simulink model "supercaps_dcbus_control"  (Simulink 7.2)
settings: Solver=ode45  StartTime=0.0  StopTime=5  RelTol=1e-5
undefined symbols (not defined in the file): C_dc, C_sto, K_i, K_v, L, T_i, T_v, V_dc0, V_dc_set, V_sto0
libraries: simulink x3
settings Model: Creator=Pierre  LastModifiedBy=Pierre

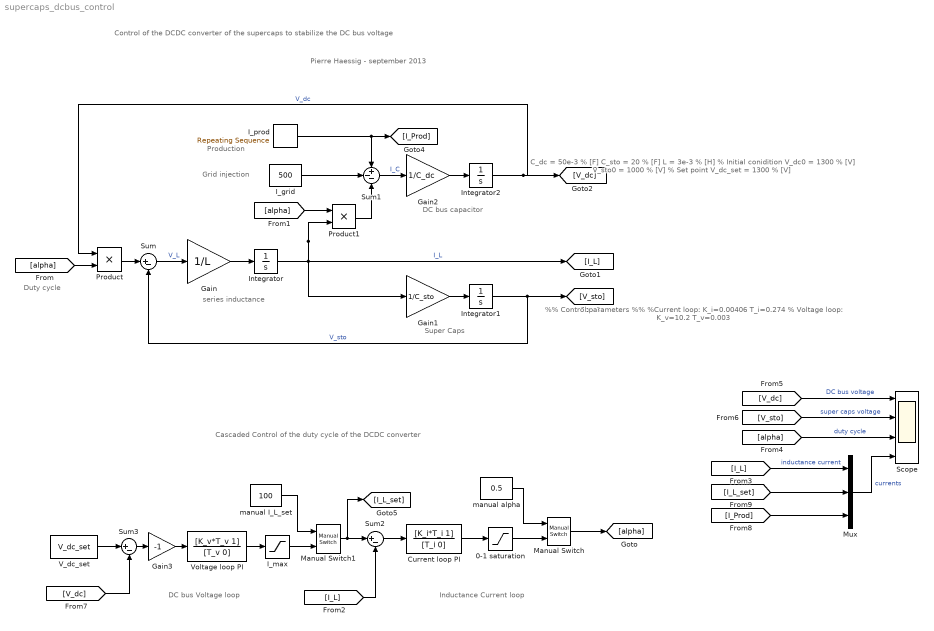
== system supercaps_dcbus_control ==
  note: Control of the DCDC converter of the supercaps
      | to stabilize the DC bus voltage
  note: Production
  note: C_dc = 50e-3 % [F]
      | C_sto = 20 % [F]
      | L = 3e-3 % [H]
      |
      | % Initial conidition
      | V_dc0 = 1300 % [V]
      | V_sto0 = 1000 % [V]
      |
      | % Set point
      | V_dc_set = 1300 % [V]
  note: Grid injection
  note: Cascaded Control
      | of the duty cycle of the DCDC converter
  note: DC bus capacitor
  note: Super Caps
  note: series inductance
  note: Pierre Haessig - september 2013
  note: %% Control parameters %%
      | %Current loop:
      | K_i=0.00406
      | T_i=0.274
      | % Voltage loop:
      | K_v=10.2
      | T_v=0.003
  note: Duty cycle
  note: DC bus Voltage loop
  note: Inductance Current loop
  0-1 saturation : Saturate  UpperLimit=1  LowerLimit=0  OutDataType=sfix(16)  OutScaling=2^0
  Current loop PI : TransferFcn  Numerator=[K_i*T_i 1]  Denominator=[T_i 0]
  Gain : Gain  Gain=1/L  ParameterDataType=sfix(16)  ParameterScaling=2^0  OutDataType=sfix(16)  OutScaling=2^0
  Gain1 : Gain  Gain=1/C_sto  ParameterDataType=sfix(16)  ParameterScaling=2^0  OutDataType=sfix(16)  OutScaling=2^0
  Gain2 : Gain  Gain=1/C_dc  ParameterDataType=sfix(16)  ParameterScaling=2^0  OutDataType=sfix(16)  OutScaling=2^0
  Gain3 : Gain  Gain=-1  ParameterDataType=sfix(16)  ParameterScaling=2^0  OutDataType=sfix(16)  OutScaling=2^0
  I_grid : Constant  Value=500  OutDataType=sfix(16)  OutScaling=2^0
  I_max : Saturate  UpperLimit=1000  LowerLimit=-1000  OutDataType=sfix(16)  OutScaling=2^0
  I_prod : simulink/Sources/Repeating Sequence  SystemSampleTime=-1  rep_seq_t=[0 2 4]  rep_seq_y=[0 1000 0]
  Integrator : Integrator
  Integrator1 : Integrator  InitialCondition=V_sto0
  Integrator2 : Integrator  InitialCondition=V_dc0
  Manual Switch : simulink/Signal Routing/Manual Switch  SystemSampleTime=-1  sw=0  action=0  varsize=off
  Manual Switch1 : simulink/Signal Routing/Manual Switch  SystemSampleTime=-1  sw=0  action=0  varsize=off
  Mux : Mux  Inputs=3
  Product : Product  OutDataType=sfix(16)  OutScaling=2^0  RndMeth=Zero
  Product1 : Product  OutDataType=sfix(16)  OutScaling=2^0  RndMeth=Zero
  Scope : Scope  NumInputPorts=4
      settings: TimeRange=10  YMin=1000~960~-0.5~-4000  YMax=3000~1040~1.5~4000
  Sum : Sum  Inputs=|+-  OutDataType=sfix(16)  OutScaling=2^0
  Sum1 : Sum  Inputs=+--  OutDataType=sfix(16)  OutScaling=2^0
  Sum2 : Sum  Inputs=|+-  OutDataType=sfix(16)  OutScaling=2^0
  Sum3 : Sum  Inputs=|+-  OutDataType=sfix(16)  OutScaling=2^0
  V_dc_set : Constant  Value=V_dc_set  OutDataType=sfix(16)  OutScaling=2^0
  Voltage loop PI : TransferFcn  Numerator=[K_v*T_v 1]  Denominator=[T_v 0]
  manual I_L_set : Constant  Value=100  OutDataType=sfix(16)  OutScaling=2^0
  manual alpha : Constant  Value=0.5  OutDataType=sfix(16)  OutScaling=2^0
  wires:
  Gain/1 -> Integrator/1
  Gain1/1 -> Integrator1/1
  Gain2/1 -> Integrator2/1
  Integrator1/1 -> Sum/2, [V_sto]  "V_sto"
  Sum/1 -> Gain/1  "V_L"
  Product/1 -> Sum/1
  Integrator2/1 -> Product/1, [V_dc]  "V_dc"
  I_prod/1 -> Sum1/1, [I_Prod]
  I_grid/1 -> Sum1/2
  [alpha] -> Product/2
  [alpha] -> Product1/1
  Product1/1 -> Sum1/3
  Sum1/1 -> Gain2/1  "I_C"
  Integrator/1 -> Gain1/1, Product1/2, [I_L]  "I_L"
  Current loop PI/1 -> 0-1 saturation/1
  [I_L] -> Sum2/2
  Sum2/1 -> Current loop PI/1
  [V_dc] -> Scope/1  "DC bus voltage"
  [V_sto] -> Scope/2  "super caps voltage"
  [alpha] -> Scope/3  "duty cycle"
  V_dc_set/1 -> Sum3/1
  [V_dc] -> Sum3/2
  0-1 saturation/1 -> Manual Switch/2
  Manual Switch/1 -> [alpha]
  manual alpha/1 -> Manual Switch/1
  Manual Switch1/1 -> Sum2/1, [I_L_set]
  manual I_L_set/1 -> Manual Switch1/1
  Mux/1 -> Scope/4  "currents"
  [I_Prod] -> Mux/3
  [I_L] -> Mux/1  "inductance current"
  [I_L_set] -> Mux/2
  Voltage loop PI/1 -> I_max/1
  I_max/1 -> Manual Switch1/2
  Sum3/1 -> Gain3/1
  Gain3/1 -> Voltage loop PI/1
